simulink model "ModParameters"  (R2019a)
settings: Solver=VariableStepAuto  StartTime=0.0  StopTime=length(Vbat.signals.values)/1000-1/1000  RelTol=1e-3
undefined symbols (not defined in the file): DiscIntNeverNeededParam
settings Model: Creator=danis  LastModifiedBy=danis

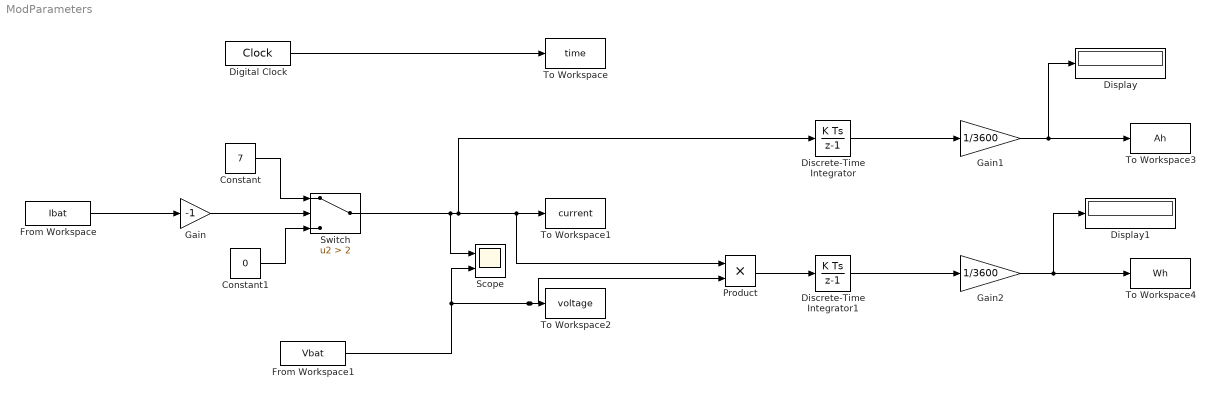
== system ModParameters ==
  Constant : Constant  Value=7  SampleTime=0.001
  Constant1 : Constant  Value=0  SampleTime=0.001
  Digital Clock : DigitalClock  SampleTime=0.001
  Discrete-Time Integrator : DiscreteIntegrator  SampleTime=-1  ICPrevOutput=DiscIntNeverNeededParam  ICPrevScaledInput=DiscIntNeverNeededParam
  Discrete-Time Integrator1 : DiscreteIntegrator  SampleTime=-1  ICPrevOutput=DiscIntNeverNeededParam  ICPrevScaledInput=DiscIntNeverNeededParam
  Display : Display
  Display1 : Display
  From Workspace : FromWorkspace  VariableName=Ibat  SampleTime=0.001  Interpolate=off  OutputAfterFinalValue=Cyclic repetition
  From Workspace1 : FromWorkspace  VariableName=Vbat  SampleTime=0.001  Interpolate=off  OutputAfterFinalValue=Cyclic repetition
  Gain : Gain  Gain=-1
  Gain1 : Gain  Gain=1/3600
  Gain2 : Gain  Gain=1/3600
  Product : Product
  Scope : Scope  NumInputPorts=2
  Switch : Switch  Criteria=u2 > Threshold  Threshold=2
  To Workspace : ToWorkspace  VariableName=time  SampleTime=-1
  To Workspace1 : ToWorkspace  VariableName=current  SampleTime=-1
  To Workspace2 : ToWorkspace  VariableName=voltage  SampleTime=-1
  To Workspace3 : ToWorkspace  VariableName=Ah  SampleTime=-1
  To Workspace4 : ToWorkspace  VariableName=Wh  SampleTime=-1
  wires:
  Digital Clock/1 -> To Workspace/1
  From Workspace/1 -> Gain/1
  From Workspace1/1 -> Product/2, To Workspace2/1, Scope/2
  Discrete-Time Integrator/1 -> Gain1/1
  Gain1/1 -> To Workspace3/1, Display/1
  Product/1 -> Discrete-Time Integrator1/1
  Discrete-Time Integrator1/1 -> Gain2/1
  Gain2/1 -> To Workspace4/1, Display1/1
  Constant/1 -> Switch/1
  Constant1/1 -> Switch/3
  Gain/1 -> Switch/2
  Switch/1 -> Scope/1, Discrete-Time Integrator/1, Product/1, To Workspace1/1
